simulink library "vs"  (Simulink 5.0)
values from neighbouring files (symbols this model uses):
  RPY = tr2rpy(T0c)    [slidevar.m]
undefined symbols (not defined in the file or in its folder): CamView, ContrLaw
libraries: simulink x24, simulink3 x23, vs x8, vs1 x1
settings Model: LastModifiedBy=ecervera

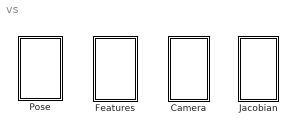
== system vs ==
  Camera : Subsystem
  Features : Subsystem
  Jacobian : Subsystem
  Pose : Subsystem

== system vs/Camera ==
  Camera view : Subsystem  LoadFcn=CamView([],[],[],'LoadBlock')  StartFcn=CamView([],[],[],'Start')  StopFcn=CamView([],[],[],'Stop')  mask{ms=15, em=normal, umin=0, umax=511, vmin=0, vmax=511, st=-1}
      mask prompts: ms "Marker Size"; em "Erase Mode"; st "Sample time"
      settings: CopyFcn=CamView([],[],[],'CopyBlock')  DeleteFcn=CamView([],[],[],'DeleteBlock')  NameChangeFcn=CamView([],[],[],'NameChange')
      mask StyleString: edit,popup(normal|none),edit,edit,edit,edit,edit
  Image of RSP : Subsystem  mask{fu=1, fv=1, u0=0, v0=0}
      mask help: Camera projection of a rigid set of points in camera frame.
  Pose estimation : Subsystem  mask{fu=1000, fv=1000, u0=256, v0=256, threshold=0.001}

== system vs/Features ==
  DTrans : Subsystem
  ITrans : Subsystem
  Penta object : vs/Features/Rigid Set of Points  x=[0 0.25 0.25 -0.25 -0.25]  y=[0 -0.25 0.25 0.25 -0.25]  z=[0 0 0 0 0]
  Point Matrix : Subsystem  mask{m=[]}
      mask prompts: m "Point Matrix (4 x N)"
      mask help: Homogeneous coordinates of a set of 3D points (each point is a matrix column).
  Quad object : vs/Features/Rigid Set of Points  x=[0.25 0.25 -0.25 -0.25]  y=[-0.25 0.25 0.25 -0.25]  z=[0 0 0 0]
  Rigid Set of Points : Subsystem  mask{x=[], y=[], z=[]}
      mask prompts: x "X-vector"; y "Y-vector"; z "Z-vector"
      mask help: Homogeneous coordinates of a set of 3D points (each point is a matrix column).
  Z's of RSP : Subsystem

== system vs/Jacobian ==
  Hand-coded control law : Subsystem  mask{n=5, fu=1000, fv=1000, u0=256, v0=256, lambda=0.125}
      mask prompts: n "Number of points"
  Inverse J : Subsystem
  Jacobian  of 2D points : Subsystem  mask{fu=1000, fv=1000, u0=256, v0=256, lambda=1}
      mask prompts: lambda "Gain"
      mask help: Converts a matrix of pixels (u,v) to a feature vector s of points (x,y) with focal=1.
  Jacobian of 3D points : Subsystem
  Jacobian of RSP : Subsystem
  PBcontrol : Subsystem  mask{lambda=0.05}
      mask prompts: lambda "Gain (>0)"
  PI control law : Subsystem  mask{lambda=1, mu=}
      mask prompts: lambda "Proportional gain (>0)"; mu "Integral gain (>0)"
      mask help: Computes the kinematic screw V = - gain J+ (s - s*).
  Pixel2s : Subsystem  mask{fu=, fv=, u0=, v0=}
      mask help: Converts a matrix of pixels (u,v) to a feature vector s of points (x,y) with focal=1.
  Proportional control law : Subsystem  mask{lambda=1}
      mask prompts: lambda "Gain (>0)"
      mask help: Computes the kinematic screw V = - gain J+ (s - s*).
  Rank J : Subsystem
  Target feature : Subsystem  mask{s=[]}
      mask prompts: s "s*"
      mask help: Column vector of target features: [s1; s2; s3; .... ; sn].
  s for points 3D : Subsystem

== system vs/Pose ==
  Composition : Subsystem
  Frame motion : Subsystem
  Inverse : Subsystem
  Pose : Subsystem  mask{x=0, y=0, z=0, r=RPY, phi=0, theta=0, psi=0}
      mask prompts: r "Rotation"
      mask help: Transformation of a translation + rotation.
      mask StyleString: edit,edit,edit,popup(RPY|Euler),edit,edit,edit
  Pose2Putheta : Subsystem
  Relative : Subsystem
  ScrewTrMat : Subsystem
  ScrewTrans : Subsystem
  skew-sym : Subsystem

== system vs/Camera/Camera view ==
  uv : Inport
  Reshape : simulink3/Signals & Systems/Reshape  OutputDimensionality=1-D array  OutputDimensions=[1,1]
  S-Function : S-Function  FunctionName=CamView  Parameters=[umin umax vmin vmax],st,ms,em
  wires:
  Reshape/1 -> S-Function/1
  uv/1 -> Reshape/1

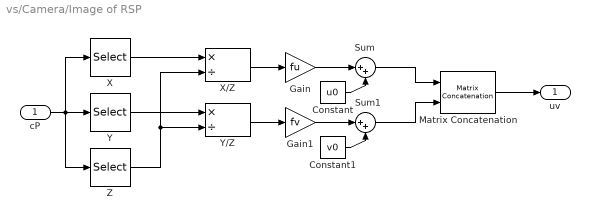
== system vs/Camera/Image of RSP ==
  cP : Inport
  Constant : Constant  Value=u0
  Constant1 : Constant  Value=v0
  Gain : Gain  Gain=fu  SaturateOnIntegerOverflow=on
  Gain1 : Gain  Gain=fv  SaturateOnIntegerOverflow=on
  Matrix Concatenation : simulink3/Signals & Systems/Matrix Concatenation  numInports=2  catMethod=Vertical
  Sum : Sum  Inputs=|++  SaturateOnIntegerOverflow=on  InputSameDT=on
  Sum1 : Sum  Inputs=|++  SaturateOnIntegerOverflow=on  InputSameDT=on
  X : Selector  InputType=Matrix  Elements=[1 3]  Columns=-1  InputPortWidth=3
  X/Z : Product  Inputs=*/  SaturateOnIntegerOverflow=on  InputSameDT=on
  Y : Selector  InputType=Matrix  Elements=[1 3]  Rows=2  Columns=-1  InputPortWidth=3
  Y/Z : Product  Inputs=*/  SaturateOnIntegerOverflow=on  InputSameDT=on
  Z : Selector  InputType=Matrix  Elements=[1 3]  Rows=3  Columns=-1  InputPortWidth=3
  uv : Outport
  wires:
  cP/1 -> X/1, Y/1, Z/1
  X/1 -> X/Z/1
  Z/1 -> X/Z/2, Y/Z/2
  Y/1 -> Y/Z/1
  Y/Z/1 -> Gain1/1
  X/Z/1 -> Gain/1
  Gain/1 -> Sum/1
  Gain1/1 -> Sum1/1
  Constant/1 -> Sum/2
  Constant1/1 -> Sum1/2
  Sum/1 -> Matrix Concatenation/1
  Sum1/1 -> Matrix Concatenation/2
  Matrix Concatenation/1 -> uv/1

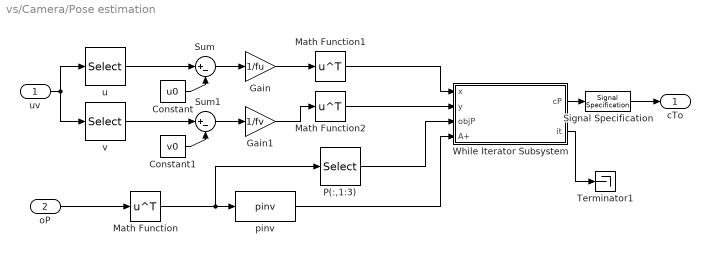
== system vs/Camera/Pose estimation ==
  uv : Inport
  oP : Inport  Port=2
  Constant : Constant  Value=u0
  Constant1 : Constant  Value=v0
  Gain : Gain  Gain=1/fu  SaturateOnIntegerOverflow=on
  Gain1 : Gain  Gain=1/fv  SaturateOnIntegerOverflow=on
  Math Function : Math  Operator=transpose
  Math Function1 : Math  Operator=transpose
  Math Function2 : Math  Operator=transpose
  P(:,1:3) : Selector  InputType=Matrix  Elements=[1 3]  Rows=-1  Columns=[1 2 3]  InputPortWidth=3
  Signal Specification : simulink/Signal Attributes/Signal Specification  D=[4 4]  Ts=-1  DataType=auto  OutDataType=sfix(16)  OutScaling=2^0
      settings: SignalType=auto  SamplingMode=auto
  Sum : Sum  Inputs=|+-  SaturateOnIntegerOverflow=on  InputSameDT=on
  Sum1 : Sum  Inputs=|+-  SaturateOnIntegerOverflow=on  InputSameDT=on
  Terminator1 : Terminator
  While Iterator Subsystem : Subsystem  TreatAsAtomicUnit=on
  pinv : MATLABFcn  MATLABFcn=pinv  Output1D=off
  u : Selector  InputType=Matrix  Elements=[1 3]  Columns=-1  InputPortWidth=3
  v : Selector  InputType=Matrix  Elements=[1 3]  Rows=2  Columns=-1  InputPortWidth=3
  cTo : Outport
  wires:
  While Iterator Subsystem/1(cP) -> Signal Specification/1
  uv/1 -> u/1, v/1
  u/1 -> Sum/1
  v/1 -> Sum1/1
  Constant/1 -> Sum/2
  Constant1/1 -> Sum1/2
  Sum/1 -> Gain/1
  Sum1/1 -> Gain1/1
  Gain/1 -> Math Function1/1
  Gain1/1 -> Math Function2/1
  oP/1 -> Math Function/1
  Math Function/1 -> pinv/1, P(:,1:3)/1
  Math Function1/1 -> While Iterator Subsystem/1(x)
  pinv/1 -> While Iterator Subsystem/4(A+)
  Math Function2/1 -> While Iterator Subsystem/2(y)
  P(:,1:3)/1 -> While Iterator Subsystem/3(objP)
  While Iterator Subsystem/2(it) -> Terminator1/1
  Signal Specification/1 -> cTo/1

== system vs/Features/DTrans ==
  aTb : Inport
  bP : Inport  Port=2
  Product : Product  Multiplication=Matrix(*)  SaturateOnIntegerOverflow=on  InputSameDT=on
  aP : Outport
  wires:
  aTb/1 -> Product/1
  bP/1 -> Product/2
  Product/1 -> aP/1

== system vs/Features/ITrans ==
  aTb : Inport
  aP : Inport  Port=2
  Inverse : vs/Pose/Inverse
      settings: RTWFcnNameOpts=Auto  RTWFileNameOpts=Auto
  Product : Product  Multiplication=Matrix(*)  SaturateOnIntegerOverflow=on  InputSameDT=on
  bP : Outport
  wires:
  aP/1 -> Product/2
  Product/1 -> bP/1
  aTb/1 -> Inverse/1
  Inverse/1 -> Product/1

== system vs/Features/Point Matrix ==
  Constant : Constant  Value=m  VectorParams1D=off
  P : Outport
  wires:
  Constant/1 -> P/1

== system vs/Features/Rigid Set of Points ==
  Constant : Constant  Value=[x;y;z;ones(1,length(x))]  VectorParams1D=off
  P : Outport
  wires:
  Constant/1 -> P/1

== system vs/Features/Z's of RSP ==
  P : Inport
  Math Function : Math  Operator=transpose
  Select Z : Selector  InputType=Matrix  Elements=[1 3]  Rows=3  Columns=-1  InputPortWidth=3
  Z : Outport
  wires:
  P/1 -> Select Z/1
  Select Z/1 -> Math Function/1
  Math Function/1 -> Z/1

== system vs/Jacobian/Hand-coded control law ==
  uv : Inport
  Z : Inport  Port=2
  uv* : Inport  Port=3
  MATLAB Fcn : MATLABFcn  MATLABFcn=ContrLaw(reshape(u(1:2*n),2,n),u(2*n+1:3*n),reshape(u(3*n+1:5*n),2,n),fu,fv,u0,v0,lambda)  OutputDimensions=6  Output1D=off
  Mux : Mux  Inputs=3
  Reshape : simulink3/Signals & Systems/Reshape  OutputDimensionality=1-D array  OutputDimensions=[1,1]
  Reshape1 : simulink3/Signals & Systems/Reshape  OutputDimensionality=1-D array  OutputDimensions=[1,1]
  Reshape2 : simulink3/Signals & Systems/Reshape  OutputDimensionality=1-D array  OutputDimensions=[1,1]
  Reshape3 : simulink3/Signals & Systems/Reshape  OutputDimensionality=Column vector  OutputDimensions=[1,1]
  cVc : Outport
  wires:
  MATLAB Fcn/1 -> Reshape3/1
  uv/1 -> Reshape/1
  Z/1 -> Reshape1/1
  uv*/1 -> Reshape2/1
  Mux/1 -> MATLAB Fcn/1
  Reshape/1 -> Mux/1
  Reshape1/1 -> Mux/2
  Reshape2/1 -> Mux/3
  Reshape3/1 -> cVc/1

== system vs/Jacobian/Inverse J ==
  J : Inport
  pinv : MATLABFcn  MATLABFcn=pinv  Output1D=off
  J+ : Outport
  wires:
  J/1 -> pinv/1
  pinv/1 -> J+/1

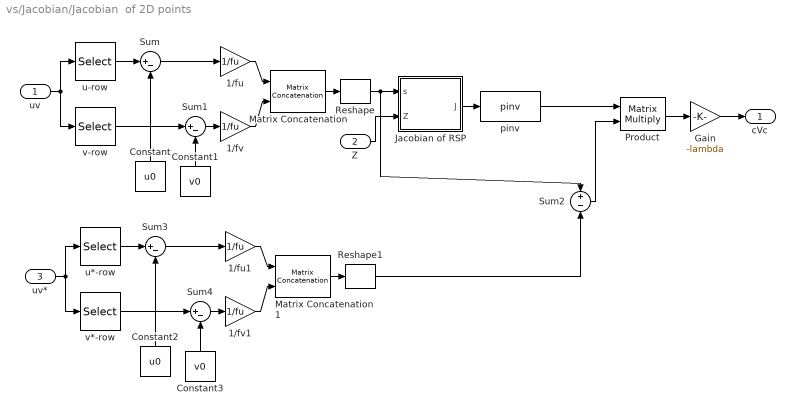
== system vs/Jacobian/Jacobian  of 2D points ==
  uv : Inport
  Z : Inport  Port=2
  uv* : Inport  Port=3
  1/fu : Gain  Gain=1/fu  SaturateOnIntegerOverflow=on
  1/fu1 : Gain  Gain=1/fu  SaturateOnIntegerOverflow=on
  1/fv : Gain  Gain=1/fu  SaturateOnIntegerOverflow=on
  1/fv1 : Gain  Gain=1/fu  SaturateOnIntegerOverflow=on
  Constant : Constant  Orientation=up  Value=u0
  Constant1 : Constant  Orientation=up  Value=v0
  Constant2 : Constant  Orientation=up  Value=u0
  Constant3 : Constant  Orientation=up  Value=v0
  Gain : Gain  Gain=-lambda  SaturateOnIntegerOverflow=on
  Jacobian of RSP : Subsystem
  Matrix Concatenation : simulink3/Signals & Systems/Matrix Concatenation  numInports=2  catMethod=Vertical
  Matrix Concatenation1 : simulink3/Signals & Systems/Matrix Concatenation  numInports=2  catMethod=Vertical
  Product : Product  Multiplication=Matrix(*)  SaturateOnIntegerOverflow=on  InputSameDT=on
  Reshape : simulink3/Signals & Systems/Reshape  OutputDimensionality=Column vector  OutputDimensions=[1,1]
  Reshape1 : simulink3/Signals & Systems/Reshape  OutputDimensionality=Column vector  OutputDimensions=[1,1]
  Sum{,1,3..4} (4 alike) : Sum  Inputs=|+-  SaturateOnIntegerOverflow=on  InputSameDT=on
  Sum2 : Sum  Inputs=+-  SaturateOnIntegerOverflow=on  InputSameDT=on
  pinv : MATLABFcn  MATLABFcn=pinv  Output1D=off
  u*-row : Selector  InputType=Matrix  Elements=[1 3]  Columns=-1  InputPortWidth=3
  u-row : Selector  InputType=Matrix  Elements=[1 3]  Columns=-1  InputPortWidth=3
  v*-row : Selector  InputType=Matrix  Elements=[1 3]  Rows=2  Columns=-1  InputPortWidth=3
  v-row : Selector  InputType=Matrix  Elements=[1 3]  Rows=2  Columns=-1  InputPortWidth=3
  cVc : Outport
  wires:
  Reshape/1 -> Jacobian of RSP/1(s), Sum2/1
  uv/1 -> v-row/1, u-row/1
  u-row/1 -> Sum/1
  v-row/1 -> Sum1/1
  Sum/1 -> 1/fu/1
  Sum1/1 -> 1/fv/1
  1/fu/1 -> Matrix Concatenation/1
  1/fv/1 -> Matrix Concatenation/2
  Matrix Concatenation/1 -> Reshape/1
  Constant/1 -> Sum/2
  Constant1/1 -> Sum1/2
  Z/1 -> Jacobian of RSP/2(Z)
  Jacobian of RSP/1(J) -> pinv/1
  Sum2/1 -> Product/2
  Product/1 -> Gain/1
  Gain/1 -> cVc/1
  pinv/1 -> Product/1
  uv*/1 -> v*-row/1, u*-row/1
  u*-row/1 -> Sum3/1
  v*-row/1 -> Sum4/1
  Sum3/1 -> 1/fu1/1
  Sum4/1 -> 1/fv1/1
  1/fu1/1 -> Matrix Concatenation1/1
  1/fv1/1 -> Matrix Concatenation1/2
  Matrix Concatenation1/1 -> Reshape1/1
  Constant2/1 -> Sum3/2
  Constant3/1 -> Sum4/2
  Reshape1/1 -> Sum2/2

== system vs/Jacobian/Jacobian of 3D points ==
  s : Inport
  Constant : Constant  Value=3
  Jacobian stack : Subsystem  TreatAsAtomicUnit=on
  Product : Product  Inputs=*/  SaturateOnIntegerOverflow=on  InputSameDT=on
  Width : Width
  J : Outport
  wires:
  Jacobian stack/1(J) -> J/1
  s/1 -> Jacobian stack/1(s), Width/1
  Product/1 -> Jacobian stack/2(n)
  Width/1 -> Product/1
  Constant/1 -> Product/2

== system vs/Jacobian/Jacobian of RSP ==
  s : Inport
  Z : Inport  Port=2
  Jacobian stack : Subsystem  TreatAsAtomicUnit=on
  Width : Width
  J : Outport
  wires:
  Jacobian stack/1(J) -> J/1
  s/1 -> Jacobian stack/1(s)
  Width/1 -> Jacobian stack/3(n)
  Z/1 -> Width/1, Jacobian stack/2(Z)

== system vs/Jacobian/PBcontrol ==
  P : Inport
  u : Inport  Port=2
  theta : Inport  Port=3
  Gain : Gain  Gain=lambda  SaturateOnIntegerOverflow=on
  Matrix Concatenation : simulink3/Signals & Systems/Matrix Concatenation  numInports=2  catMethod=Vertical
  Product : Product  SaturateOnIntegerOverflow=on  InputSameDT=on
  cVc : Outport
  wires:
  Product/1 -> Matrix Concatenation/2
  Matrix Concatenation/1 -> Gain/1
  P/1 -> Matrix Concatenation/1
  u/1 -> Product/1
  Gain/1 -> cVc/1
  theta/1 -> Product/2

== system vs/Jacobian/PI control law ==
  J+ : Inport
  s : Inport  Port=2
  s* : Inport  Port=3
  Gain : Gain  Gain=-lambda  SaturateOnIntegerOverflow=on
  Gain1 : Gain  Gain=-mu  SaturateOnIntegerOverflow=on
  Integrator : Integrator
  Product : Product  Multiplication=Matrix(*)  SaturateOnIntegerOverflow=on  InputSameDT=on
  Sum : Sum  Inputs=+-  SaturateOnIntegerOverflow=on  InputSameDT=on
  Sum1 : Sum  Inputs=|++  SaturateOnIntegerOverflow=on  InputSameDT=on
  cVc : Outport
  wires:
  s/1 -> Sum/1
  s*/1 -> Sum/2
  J+/1 -> Product/1
  Sum/1 -> Product/2
  Product/1 -> Gain/1, Integrator/1
  Integrator/1 -> Gain1/1
  Gain/1 -> Sum1/1
  Sum1/1 -> cVc/1
  Gain1/1 -> Sum1/2

== system vs/Jacobian/Pixel2s ==
  uv : Inport
  1/fu : Gain  Gain=1/fu  SaturateOnIntegerOverflow=on
  1/fv : Gain  Gain=1/fu  SaturateOnIntegerOverflow=on
  Constant : Constant  Orientation=up  Value=u0
  Constant1 : Constant  Orientation=up  Value=v0
  Matrix Concatenation : simulink3/Signals & Systems/Matrix Concatenation  numInports=2  catMethod=Vertical
  Reshape : simulink3/Signals & Systems/Reshape  OutputDimensionality=Column vector  OutputDimensions=[1,1]
  Sum : Sum  Inputs=|+-  SaturateOnIntegerOverflow=on  InputSameDT=on
  Sum1 : Sum  Inputs=|+-  SaturateOnIntegerOverflow=on  InputSameDT=on
  u-row : Selector  InputType=Matrix  Elements=[1 3]  Columns=-1  InputPortWidth=3
  v-row : Selector  InputType=Matrix  Elements=[1 3]  Rows=2  Columns=-1  InputPortWidth=3
  s : Outport
  wires:
  Reshape/1 -> s/1
  uv/1 -> v-row/1, u-row/1
  u-row/1 -> Sum/1
  v-row/1 -> Sum1/1
  Sum/1 -> 1/fu/1
  Sum1/1 -> 1/fv/1
  1/fu/1 -> Matrix Concatenation/1
  1/fv/1 -> Matrix Concatenation/2
  Matrix Concatenation/1 -> Reshape/1
  Constant/1 -> Sum/2
  Constant1/1 -> Sum1/2

== system vs/Jacobian/Proportional control law ==
  J+ : Inport
  s : Inport  Port=2
  s* : Inport  Port=3
  Gain : Gain  Gain=-lambda  SaturateOnIntegerOverflow=on
  Product : Product  Multiplication=Matrix(*)  SaturateOnIntegerOverflow=on  InputSameDT=on
  Sum : Sum  Inputs=+-  SaturateOnIntegerOverflow=on  InputSameDT=on
  cVc : Outport
  wires:
  s/1 -> Sum/1
  s*/1 -> Sum/2
  J+/1 -> Product/1
  Sum/1 -> Product/2
  Product/1 -> Gain/1
  Gain/1 -> cVc/1

== system vs/Jacobian/Rank J ==
  J : Inport
  rank : MATLABFcn  MATLABFcn=rank  Output1D=off
  Rank(J) : Outport
  wires:
  J/1 -> rank/1
  rank/1 -> Rank(J)/1

== system vs/Jacobian/Target feature ==
  Constant : Constant  Value=s  VectorParams1D=off
  s* : Outport
  wires:
  Constant/1 -> s*/1

== system vs/Jacobian/s for points 3D ==
  cP : Inport
  Reshape : simulink3/Signals & Systems/Reshape  OutputDimensionality=Column vector  OutputDimensions=[1,1]
  Selector : Selector  InputType=Matrix  Elements=[1 3]  Rows=[1 2 3]  Columns=-1  InputPortWidth=3
  s : Outport
  wires:
  cP/1 -> Selector/1
  Reshape/1 -> s/1
  Selector/1 -> Reshape/1

== system vs/Pose/Composition ==
  aTb : Inport
  bTc : Inport  Port=2
  Product : Product  Multiplication=Matrix(*)  SaturateOnIntegerOverflow=on  InputSameDT=on
  aTc : Outport
  wires:
  Product/1 -> aTc/1
  aTb/1 -> Product/1
  bTc/1 -> Product/2

== system vs/Pose/Frame motion ==
  iTj(0) : Inport
  jVj : Inport  Port=2
  Differential : Subsystem
  Motion : Subsystem
  iTj(t) : Outport
  wires:
  Differential/1(diTj) -> Motion/2(diTj)
  iTj(0)/1 -> Motion/1(iTj(0))
  Motion/1(iTj(t)) -> iTj(t)/1, Differential/1(iTj)
  jVj/1 -> Differential/2(Vj)

== system vs/Pose/Inverse ==
  aTb : Inport
  Math Function : Math  Operator=transpose
  Matrix Gain : Gain  Gain=[1 0 0 0; 0 1 0 0; 0 0 1 0; 0 0 0 -1]  Multiplication=Matrix(u*K)  SaturateOnIntegerOverflow=on
  Matrix Gain1 : Gain  Gain=[1 0 0 0; 0 1 0 0; 0 0 1 0; 0 0 0 -1]  Multiplication=Matrix(u*K)  SaturateOnIntegerOverflow=on
  Product1 : Product  Multiplication=Matrix(*)  SaturateOnIntegerOverflow=on  InputSameDT=on
  Split : Subsystem
  bTa : Outport
  wires:
  aTb/1 -> Split/1(T)
  Split/1(R) -> Math Function/1
  Product1/1 -> bTa/1
  Matrix Gain/1 -> Product1/2
  Split/2(P) -> Matrix Gain/1
  Matrix Gain1/1 -> Product1/1
  Math Function/1 -> Matrix Gain1/1

== system vs/Pose/Pose ==
  Constant : Constant  Value=r
  Euler-rotation : Subsystem  mask{phi=phi, theta=theta, psi=psi}
      mask help: Transformation of a rotation specified by Euler angles: T = rot(z,phi) rot(x,theta) rot(z, psi).
  Product : Product  Multiplication=Matrix(*)  SaturateOnIntegerOverflow=on  InputSameDT=on
  RPY-rotation : Subsystem  mask{phi=phi, theta=theta, psi=psi}
      mask help: Transformation of a rotation specified by Euler angles: T = rot(z,phi) rot(x,theta) rot(z, psi).
  Switch : Switch  Threshold=1.5  SaturateOnIntegerOverflow=on  InputSameDT=on
  Translation : Subsystem  mask{x=x, y=y, z=z}
      mask help: Transformation of a pure translation.
  T : Outport
  wires:
  Euler-rotation/1(T) -> Switch/1
  RPY-rotation/1(T) -> Switch/3
  Constant/1 -> Switch/2
  Product/1 -> T/1
  Translation/1(T) -> Product/1
  Switch/1 -> Product/2

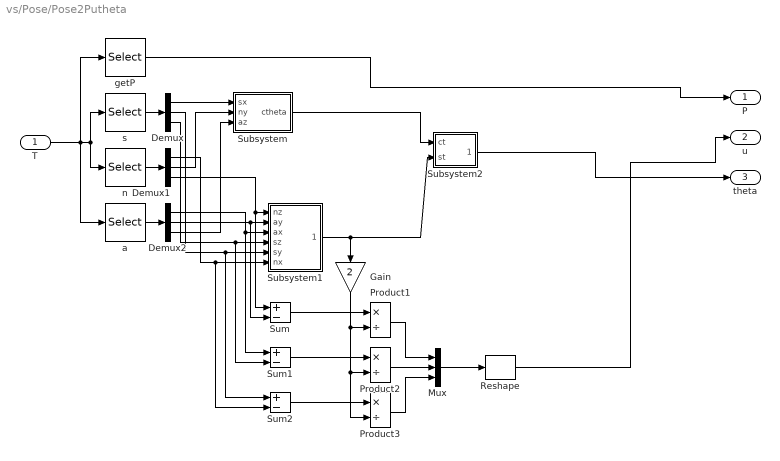
== system vs/Pose/Pose2Putheta ==
  T : Inport
  Demux : Demux  Outputs=3
  Demux1 : Demux  Outputs=3
  Demux2 : Demux  Outputs=3
  Gain : Gain  Orientation=down  Gain=2  SaturateOnIntegerOverflow=on
  Mux : Mux  Inputs=3
  Product1 : Product  Inputs=*/  SaturateOnIntegerOverflow=on  InputSameDT=on
  Product2 : Product  Inputs=*/  SaturateOnIntegerOverflow=on  InputSameDT=on
  Product3 : Product  Inputs=*/  SaturateOnIntegerOverflow=on  InputSameDT=on
  Reshape : simulink3/Signals & Systems/Reshape  OutputDimensionality=Column vector  OutputDimensions=[1,1]
  Subsystem : Subsystem
  Subsystem1 : Subsystem
  Subsystem2 : Subsystem
  Sum : Sum  Inputs=+-  SaturateOnIntegerOverflow=on  InputSameDT=on
  Sum1 : Sum  Inputs=+-  SaturateOnIntegerOverflow=on  InputSameDT=on
  Sum2 : Sum  Inputs=+-  SaturateOnIntegerOverflow=on  InputSameDT=on
  a : Selector  InputType=Matrix  Elements=[1 3]  Rows=[1 2 3]  Columns=3  InputPortWidth=3
  getP : Selector  InputType=Matrix  Elements=[1 3]  Rows=[1 2 3]  Columns=4  InputPortWidth=3
  n : Selector  InputType=Matrix  Elements=[1 3]  Rows=[1 2 3]  Columns=2  InputPortWidth=3
  s : Selector  InputType=Matrix  Elements=[1 3]  Rows=[1 2 3]  InputPortWidth=3
  P : Outport
  u : Outport  Port=2
  theta : Outport  Port=3
  wires:
  T/1 -> getP/1, s/1, n/1, a/1
  getP/1 -> P/1
  s/1 -> Demux/1
  n/1 -> Demux1/1
  a/1 -> Demux2/1
  Demux/1 -> Subsystem/1(sx)
  Demux1/2 -> Subsystem/2(ny)
  Demux2/3 -> Subsystem/3(az)
  Demux1/3 -> Subsystem1/1(nz), Sum/1
  Demux2/2 -> Subsystem1/2(ay), Sum/2
  Demux2/1 -> Subsystem1/3(ax), Sum1/1
  Demux/3 -> Subsystem1/4(sz), Sum1/2
  Demux/2 -> Subsystem1/5(sy), Sum2/1
  Demux1/1 -> Subsystem1/6(nx), Sum2/2
  Subsystem/1(ctheta) -> Subsystem2/1(ct)
  Subsystem1/1(stheta) -> Subsystem2/2(st), Gain/1
  Gain/1 -> Product1/2, Product2/2, Product3/2
  Sum/1 -> Product1/1
  Sum1/1 -> Product2/1
  Sum2/1 -> Product3/1
  Product2/1 -> Mux/2
  Product1/1 -> Mux/1
  Product3/1 -> Mux/3
  Subsystem2/1(theta) -> theta/1
  Mux/1 -> Reshape/1
  Reshape/1 -> u/1

== system vs/Pose/Relative ==
  aTb : Inport
  aTc : Inport  Port=2
  Inverse : vs1/Pose/Inverse
      settings: RTWFcnNameOpts=Auto  RTWFileNameOpts=Auto
  Product : Product  Multiplication=Matrix(*)  SaturateOnIntegerOverflow=on  InputSameDT=on
  bTc : Outport
  wires:
  Product/1 -> bTc/1
  aTb/1 -> Inverse/1
  Inverse/1 -> Product/1
  aTc/1 -> Product/2

== system vs/Pose/ScrewTrMat ==
  iTj : Inport
  0 3x3 : Constant  Value=zeros(3,3)  VectorParams1D=off
  Matrix Concatenation : simulink/Math Operations/Matrix Concatenation  numInports=2  catMethod=Horizontal
  Matrix Concatenation1 : simulink/Math Operations/Matrix Concatenation  numInports=2  catMethod=Horizontal
  Matrix Concatenation2 : simulink/Math Operations/Matrix Concatenation  numInports=2  catMethod=Vertical
  Product : Product  Multiplication=Matrix(*)  SaturateOnIntegerOverflow=on  InputSameDT=on
  Split : Subsystem
  iPj 3x1 : Selector  InputType=Matrix  Elements=[1 3]  Rows=[1 2 3]  Columns=4  InputPortWidth=3
  iRj 3x3 : Selector  InputType=Matrix  Elements=[1 3]  Rows=[1 2 3]  Columns=[1 2 3]  InputPortWidth=3
  sk(iPj) : vs/Pose/skew-sym  SimViewingDevice=off  DataTypeOverride=UseLocalSettings  MinMaxOverflowLogging=UseLocalSettings
      settings: Permissions=ReadWrite  RTWFcnNameOpts=Auto  RTWFileNameOpts=Auto
  iSTj : Outport
  wires:
  0 3x3/1 -> Matrix Concatenation1/1
  sk(iPj)/1 -> Product/1
  Product/1 -> Matrix Concatenation/2
  iRj 3x3/1 -> Matrix Concatenation1/2, Product/2, Matrix Concatenation/1
  Matrix Concatenation1/1 -> Matrix Concatenation2/2
  Matrix Concatenation/1 -> Matrix Concatenation2/1
  Matrix Concatenation2/1 -> iSTj/1
  iPj 3x1/1 -> sk(iPj)/1
  Split/2(P) -> iPj 3x1/1
  Split/1(R) -> iRj 3x3/1
  iTj/1 -> Split/1(T)

== system vs/Pose/ScrewTrans ==
  jVj : Inport
  iTj : Inport  Port=2
  Product : Product  Multiplication=Matrix(*)  SaturateOnIntegerOverflow=on  InputSameDT=on
  ScrewTrMat : vs/Pose/ScrewTrMat  SimViewingDevice=off  DataTypeOverride=UseLocalSettings  MinMaxOverflowLogging=UseLocalSettings
      settings: Permissions=ReadWrite  RTWFcnNameOpts=Auto  RTWFileNameOpts=Auto
  iVi : Outport
  wires:
  iTj/1 -> ScrewTrMat/1
  ScrewTrMat/1 -> Product/1
  jVj/1 -> Product/2
  Product/1 -> iVi/1

== system vs/Pose/skew-sym ==
  v : Inport
  Constant : Constant  Value=[0 0 0; 0 0 1; 0 -1 0]  VectorParams1D=off
  Constant1 : Constant  Value=[0 0 -1; 0 0 0; 1 0 0]  VectorParams1D=off
  Constant2 : Constant  Value=[0 1 0; -1 0 0; 0 0 0]  VectorParams1D=off
  Matrix Concatenation : simulink/Math Operations/Matrix Concatenation  numInports=3  catMethod=Horizontal
  Product : Product  Multiplication=Matrix(*)  SaturateOnIntegerOverflow=on  InputSameDT=on
  Product1 : Product  Multiplication=Matrix(*)  SaturateOnIntegerOverflow=on  InputSameDT=on
  Product2 : Product  Multiplication=Matrix(*)  SaturateOnIntegerOverflow=on  InputSameDT=on
  Signal Specification1 : simulink/Signal Attributes/Signal Specification  D=[3 1]  Ts=-1  DataType=auto  OutDataType=sfix(16)  OutScaling=2^0
      settings: SignalType=auto  SamplingMode=auto
  Signal Specification2 : simulink/Signal Attributes/Signal Specification  D=[3 1]  Ts=-1  DataType=auto  OutDataType=sfix(16)  OutScaling=2^0
      settings: SignalType=auto  SamplingMode=auto
  Signal Specification3 : simulink/Signal Attributes/Signal Specification  D=[3 1]  Ts=-1  DataType=auto  OutDataType=sfix(16)  OutScaling=2^0
      settings: SignalType=auto  SamplingMode=auto
  sk(v) : Outport
  wires:
  Signal Specification3/1 -> Matrix Concatenation/3
  Signal Specification2/1 -> Matrix Concatenation/1
  Signal Specification1/1 -> Matrix Concatenation/2
  Constant/1 -> Product/1
  v/1 -> Product/2, Product1/2, Product2/2
  Matrix Concatenation/1 -> sk(v)/1
  Product/1 -> Signal Specification2/1
  Constant1/1 -> Product1/1
  Constant2/1 -> Product2/1
  Product1/1 -> Signal Specification1/1
  Product2/1 -> Signal Specification3/1

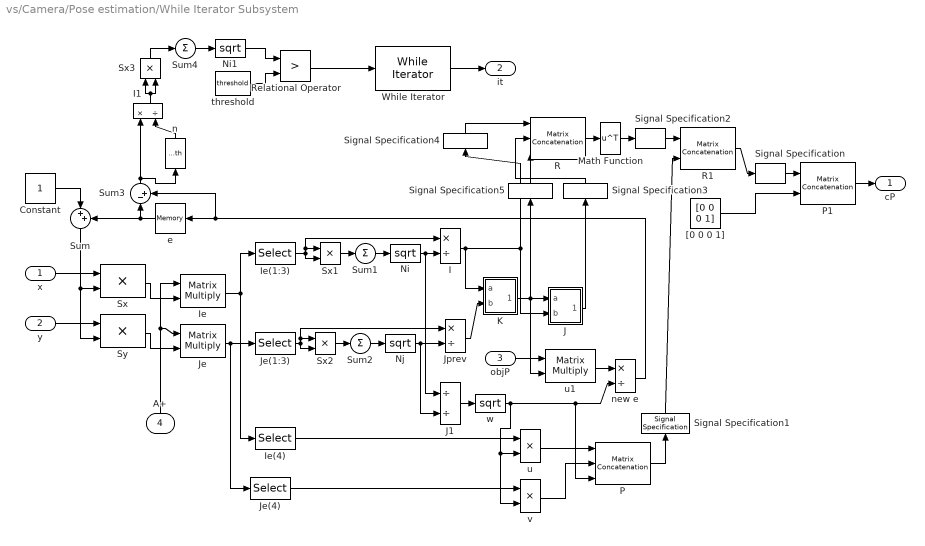
== system vs/Camera/Pose estimation/While Iterator Subsystem ==
  x : Inport
  y : Inport  Port=2
  objP : Inport  Port=3
  A+ : Inport  Orientation=up  Port=4
  Constant : Constant
  I : Product  Inputs=*/  SaturateOnIntegerOverflow=on  InputSameDT=on
  I1 : Product  Orientation=up  Inputs=*/  SaturateOnIntegerOverflow=on  InputSameDT=on
  Ie : Product  Multiplication=Matrix(*)  SaturateOnIntegerOverflow=on  InputSameDT=on
  Ie(1:3) : Selector  InputType=Matrix  Elements=[1 3]  Rows=[1 2 3]  Columns=-1  InputPortWidth=3
  Ie(4) : Selector  InputType=Matrix  Elements=[1 3]  Rows=4  Columns=-1  InputPortWidth=3
  J : Subsystem
  J1 : Product  Inputs=//  SaturateOnIntegerOverflow=on  InputSameDT=on
  Je : Product  Multiplication=Matrix(*)  SaturateOnIntegerOverflow=on  InputSameDT=on
  Je(1:3) : Selector  InputType=Matrix  Elements=[1 3]  Rows=[1 2 3]  Columns=-1  InputPortWidth=3
  Je(4) : Selector  InputType=Matrix  Elements=[1 3]  Rows=4  Columns=-1  InputPortWidth=3
  Jprev : Product  Inputs=*/  SaturateOnIntegerOverflow=on  InputSameDT=on
  K : Subsystem
  Math Function : Math  Operator=transpose
  Ni : Math  Operator=sqrt
  Ni1 : Math  Operator=sqrt
  Nj : Math  Operator=sqrt
  P : simulink/Math Operations/Matrix Concatenation  numInports=3  catMethod=Vertical
  P1 : simulink/Math Operations/Matrix Concatenation  numInports=2  catMethod=Vertical
  R : simulink/Math Operations/Matrix Concatenation  numInports=3  catMethod=Horizontal
  R1 : simulink/Math Operations/Matrix Concatenation  numInports=2  catMethod=Horizontal
  Relational Operator : RelationalOperator  Operator=>  InputSameDT=on
  Signal Specification : simulink/Signal Attributes/Signal Specification  D=[3 4]  Ts=-1  DataType=auto  OutDataType=sfix(16)  OutScaling=2^0
      settings: SignalType=auto  SamplingMode=auto
  Signal Specification{1,3..5} (4 alike) : simulink/Signal Attributes/Signal Specification  Orientation=up  D=[3 1]  Ts=-1  DataType=auto  OutDataType=sfix(16)  OutScaling=2^0
      settings: SignalType=auto  SamplingMode=auto
  Signal Specification2 : simulink/Signal Attributes/Signal Specification  D=[3 3]  Ts=-1  DataType=auto  OutDataType=sfix(16)  OutScaling=2^0
      settings: SignalType=auto  SamplingMode=auto
  Sum : Sum  Orientation=down  Inputs=|++  SaturateOnIntegerOverflow=on  InputSameDT=on
  Sum1 : Sum  Inputs=+  SaturateOnIntegerOverflow=on  InputSameDT=on
  Sum2 : Sum  Inputs=+  SaturateOnIntegerOverflow=on  InputSameDT=on
  Sum3 : Sum  Orientation=up  Inputs=|-+  SaturateOnIntegerOverflow=on  InputSameDT=on
  Sum4 : Sum  Inputs=+  SaturateOnIntegerOverflow=on  InputSameDT=on
  Sx : Product  SaturateOnIntegerOverflow=on  InputSameDT=on
  Sx1 : Product  SaturateOnIntegerOverflow=on  InputSameDT=on
  Sx2 : Product  SaturateOnIntegerOverflow=on  InputSameDT=on
  Sx3 : Product  Orientation=up  SaturateOnIntegerOverflow=on  InputSameDT=on
  Sy : Product  SaturateOnIntegerOverflow=on  InputSameDT=on
  While Iterator : WhileIterator  MaxIters=20  WhileBlockType=do-while  ShowIterationPort=on  OutputDataType=double
  "[0 0 0 1]" : Constant  Value=[0 0 0 1]  VectorParams1D=off
  e : Memory  Orientation=left  InheritSampleTime=on
  n : Width  Orientation=up
  new e : Product  Inputs=*/  SaturateOnIntegerOverflow=on  InputSameDT=on
  threshold : Constant  Value=threshold
  u : Product  Inputs=**  SaturateOnIntegerOverflow=on  InputSameDT=on
  u1 : Product  Inputs=**  Multiplication=Matrix(*)  SaturateOnIntegerOverflow=on  InputSameDT=on
  v : Product  Inputs=**  SaturateOnIntegerOverflow=on  InputSameDT=on
  w : Math  Operator=sqrt
  cP : Outport
  it : Outport  Port=2
  wires:
  x/1 -> Sx/1
  Constant/1 -> Sum/1
  Sum/1 -> Sx/2, Sy/2
  y/1 -> Sy/1
  A+/1 -> Ie/1, Je/1
  Ie/1 -> Ie(4)/1, Ie(1:3)/1
  Je/1 -> Je(1:3)/1, Je(4)/1
  Ie(1:3)/1 -> Sx1/2, Sx1/1, I/1
  Sx1/1 -> Sum1/1
  Sum1/1 -> Ni/1
  Je(1:3)/1 -> Sx2/2, Sx2/1, Jprev/1
  Sx2/1 -> Sum2/1
  Sum2/1 -> Nj/1
  Ni/1 -> I/2, J1/1
  Nj/1 -> Jprev/2, J1/2
  I/1 -> K/1(a), J/2(b), Signal Specification4/1
  Jprev/1 -> K/2(b)
  K/1(axb) -> J/1(a), u1/2, Signal Specification5/1
  J1/1 -> w/1
  Ie(4)/1 -> u/1
  w/1 -> u/2, v/2, new e/2, P/3
  Je(4)/1 -> v/1
  objP/1 -> u1/1
  u1/1 -> new e/1
  e/1 -> Sum/2, Sum3/1
  new e/1 -> e/1, Sum3/2
  Sum3/1 -> n/1, I1/1
  n/1 -> I1/2
  I1/1 -> Sx3/1, Sx3/2
  Sx3/1 -> Sum4/1
  Sum4/1 -> Ni1/1
  Ni1/1 -> Relational Operator/1
  threshold/1 -> Relational Operator/2
  Relational Operator/1 -> While Iterator/1
  While Iterator/1 -> it/1
  J/1(axb) -> Signal Specification3/1
  u/1 -> P/1
  v/1 -> P/2
  R/1 -> Math Function/1
  P/1 -> Signal Specification1/1
  R1/1 -> Signal Specification/1
  P1/1 -> cP/1
  Sx/1 -> Ie/2
  Sy/1 -> Je/2
  Math Function/1 -> Signal Specification2/1
  "[0 0 0 1]"/1 -> P1/2
  Signal Specification/1 -> P1/1
  Signal Specification1/1 -> R1/2
  Signal Specification2/1 -> R1/1
  Signal Specification3/1 -> R/2
  Signal Specification4/1 -> R/1
  Signal Specification5/1 -> R/3

== system vs/Jacobian/Jacobian  of 2D points/Jacobian of RSP ==
  s : Inport
  Z : Inport  Port=2
  Jacobian stack : Subsystem  TreatAsAtomicUnit=on
  Width : Width
  J : Outport
  wires:
  Jacobian stack/1(J) -> J/1
  s/1 -> Jacobian stack/1(s)
  Width/1 -> Jacobian stack/3(n)
  Z/1 -> Width/1, Jacobian stack/2(Z)

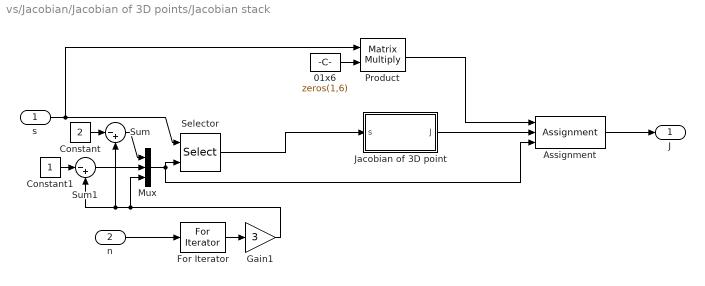
== system vs/Jacobian/Jacobian of 3D points/Jacobian stack ==
  s : Inport
  n : Inport  Port=2
  01x6 : Constant  Value=zeros(1,6)  VectorParams1D=off
  Assignment : Assignment  InputType=Matrix  RowSrc=External  Columns=-1
  Constant : Constant  Value=2
  Constant1 : Constant
  For Iterator : ForIterator  IterationSource=external  OutputDataType=double
  Gain1 : Gain  Gain=3  SaturateOnIntegerOverflow=on
  Jacobian of 3D point : Subsystem
  Mux : Mux  Inputs=3
  Product : Product  Multiplication=Matrix(*)  SaturateOnIntegerOverflow=on  InputSameDT=on
  Selector : Selector  InputType=Matrix  ElementSrc=External  Elements=[1 3]  RowSrc=External  Columns=-1  InputPortWidth=3
  Sum : Sum  Inputs=|-+  SaturateOnIntegerOverflow=on  InputSameDT=on
  Sum1 : Sum  Inputs=|-+  SaturateOnIntegerOverflow=on  InputSameDT=on
  J : Outport
  wires:
  Selector/1 -> Jacobian of 3D point/1(s)
  Jacobian of 3D point/1(J) -> Assignment/2
  Constant/1 -> Sum/1
  Sum/1 -> Mux/1
  Gain1/1 -> Mux/3, Sum/2, Sum1/2
  For Iterator/1 -> Gain1/1
  Mux/1 -> Assignment/3, Selector/2
  01x6/1 -> Product/2
  Product/1 -> Assignment/1
  Assignment/1 -> J/1
  n/1 -> For Iterator/1
  s/1 -> Selector/1, Product/1
  Constant1/1 -> Sum1/1
  Sum1/1 -> Mux/2

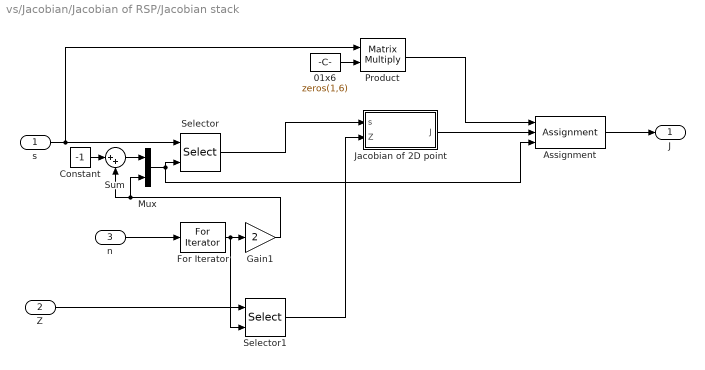
== system vs/Jacobian/Jacobian of RSP/Jacobian stack ==
  s : Inport
  Z : Inport  Port=2
  n : Inport  Port=3
  01x6 : Constant  Value=zeros(1,6)  VectorParams1D=off
  Assignment : Assignment  InputType=Matrix  RowSrc=External  Columns=-1
  Constant : Constant  Value=-1
  For Iterator : ForIterator  IterationSource=external  OutputDataType=double
  Gain1 : Gain  Gain=2  SaturateOnIntegerOverflow=on
  Jacobian of 2D point : Subsystem
  Mux : Mux  Inputs=2
  Product : Product  Multiplication=Matrix(*)  SaturateOnIntegerOverflow=on  InputSameDT=on
  Selector : Selector  InputType=Matrix  ElementSrc=External  Elements=[1 3]  RowSrc=External  Columns=-1  InputPortWidth=3
  Selector1 : Selector  InputType=Matrix  ElementSrc=External  Elements=[1 3]  RowSrc=External  Columns=-1  InputPortWidth=3
  Sum : Sum  Inputs=|++  SaturateOnIntegerOverflow=on  InputSameDT=on
  J : Outport
  wires:
  Selector1/1 -> Jacobian of 2D point/2(Z)
  Selector/1 -> Jacobian of 2D point/1(s)
  Jacobian of 2D point/1(J) -> Assignment/2
  Z/1 -> Selector1/1
  Constant/1 -> Sum/1
  Sum/1 -> Mux/1
  Gain1/1 -> Sum/2, Mux/2
  For Iterator/1 -> Selector1/2, Gain1/1
  Mux/1 -> Assignment/3, Selector/2
  01x6/1 -> Product/2
  Product/1 -> Assignment/1
  Assignment/1 -> J/1
  n/1 -> For Iterator/1
  s/1 -> Selector/1, Product/1

== system vs/Pose/Frame motion/Differential ==
  iTj : Inport
  Vj : Inport  Port=2
  Constant : Constant  Value=[0 0 0 0]  VectorParams1D=off
  Matrix Concatenation : simulink/Math Operations/Matrix Concatenation  numInports=2  catMethod=Horizontal
  Matrix Concatenation1 : simulink/Math Operations/Matrix Concatenation  numInports=2  catMethod=Vertical
  Product : Product  Multiplication=Matrix(*)  SaturateOnIntegerOverflow=on  InputSameDT=on
  Signal Specification : simulink/Signal Attributes/Signal Specification  D=[4 4]  Ts=-1  DataType=auto  OutDataType=sfix(16)  OutScaling=2^0
      settings: SignalType=auto  SamplingMode=auto
  Signal Specification1 : simulink/Signal Attributes/Signal Specification  D=[3 4]  Ts=-1  DataType=auto  OutDataType=sfix(16)  OutScaling=2^0
      settings: SignalType=auto  SamplingMode=auto
  Signal Specification2 : simulink/Signal Attributes/Signal Specification  Orientation=up  D=[3 3]  Ts=-1  DataType=auto  OutDataType=sfix(16)  OutScaling=2^0
      settings: SignalType=auto  SamplingMode=auto
  Signal Specification3 : simulink/Signal Attributes/Signal Specification  D=[3 1]  Ts=-1  DataType=auto  OutDataType=sfix(16)  OutScaling=2^0
      settings: SignalType=auto  SamplingMode=auto
  skew-sym : vs/Pose/skew-sym  SimViewingDevice=off  DataTypeOverride=UseLocalSettings  MinMaxOverflowLogging=UseLocalSettings
      settings: Permissions=ReadWrite  RTWFcnNameOpts=Auto  RTWFileNameOpts=Auto
  vj : Selector  Elements=[1 2 3]  InputPortWidth=6
  wj : Selector  Elements=[4 5 6]  InputPortWidth=6
  diTj : Outport
  wires:
  Vj/1 -> wj/1, vj/1
  wj/1 -> skew-sym/1
  skew-sym/1 -> Signal Specification2/1
  vj/1 -> Signal Specification3/1
  Matrix Concatenation/1 -> Signal Specification1/1
  Constant/1 -> Matrix Concatenation1/2
  iTj/1 -> Product/1
  Matrix Concatenation1/1 -> Product/2
  Product/1 -> Signal Specification/1
  Signal Specification/1 -> diTj/1
  Signal Specification1/1 -> Matrix Concatenation1/1
  Signal Specification2/1 -> Matrix Concatenation/1
  Signal Specification3/1 -> Matrix Concatenation/2

== system vs/Pose/Frame motion/Motion ==
  iTj(0) : Inport
  diTj : Inport  Port=2
  Integrator : Integrator
  Sum : Sum  Inputs=|++  SaturateOnIntegerOverflow=on  InputSameDT=on
  iTj(t) : Outport
  wires:
  diTj/1 -> Integrator/1
  iTj(0)/1 -> Sum/1
  Integrator/1 -> Sum/2
  Sum/1 -> iTj(t)/1

== system vs/Pose/Inverse/Split ==
  T : Inport
  GetP : Selector  InputType=Matrix  Elements=[1 3]  Rows=-1  Columns=4  InputPortWidth=3
  GetR : Selector  InputType=Matrix  Elements=[1 3]  Rows=-1  Columns=[1 2 3]  InputPortWidth=3
  Matrix Concatenation : simulink3/Signals & Systems/Matrix Concatenation  numInports=2  catMethod=Horizontal
  Matrix Concatenation1 : simulink3/Signals & Systems/Matrix Concatenation  numInports=2  catMethod=Horizontal
  P0 : Constant  Value=[0;0;0;1]  VectorParams1D=off
  RI : Constant  Value=[1 0 0; 0 1 0; 0 0 1; 0 0 0]  VectorParams1D=off
  R : Outport
  P : Outport  Port=2
  wires:
  Matrix Concatenation1/1 -> P/1
  GetP/1 -> Matrix Concatenation1/2
  RI/1 -> Matrix Concatenation1/1
  Matrix Concatenation/1 -> R/1
  P0/1 -> Matrix Concatenation/2
  GetR/1 -> Matrix Concatenation/1
  T/1 -> GetR/1, GetP/1

== system vs/Pose/Pose/Euler-rotation ==
  Product : Product  Multiplication=Matrix(*)  SaturateOnIntegerOverflow=on  InputSameDT=on
  Product1 : Product  Multiplication=Matrix(*)  SaturateOnIntegerOverflow=on  InputSameDT=on
  X-rotation theta : Subsystem  mask{phi=theta}
      mask prompts: phi "Angle"
      mask help: Transformation of a pure rotation around the x-axis.
  Z-rotation phi : Subsystem  mask{phi=phi}
      mask prompts: phi "Angle"
      mask help: Transformation of a pure rotation around the z-axis.
  Z-rotation psi : Subsystem  mask{phi=psi}
      mask prompts: phi "Angle"
      mask help: Transformation of a pure rotation around the z-axis.
  T : Outport
  wires:
  Z-rotation psi/1(T) -> Product1/2
  Product/1 -> Product1/1
  X-rotation theta/1(T) -> Product/2
  Z-rotation phi/1(T) -> Product/1
  Product1/1 -> T/1

== system vs/Pose/Pose/RPY-rotation ==
  Product : Product  Multiplication=Matrix(*)  SaturateOnIntegerOverflow=on  InputSameDT=on
  Product1 : Product  Multiplication=Matrix(*)  SaturateOnIntegerOverflow=on  InputSameDT=on
  X-rotation psi : Subsystem  mask{phi=psi}
      mask prompts: phi "Angle"
      mask help: Transformation of a pure rotation around the x-axis.
  Y-rotation theta : Subsystem  mask{phi=theta}
      mask prompts: phi "Angle"
      mask help: Transformation of a pure rotation around the y-axis.
  Z-rotation phi : Subsystem  mask{phi=phi}
      mask prompts: phi "Angle"
      mask help: Transformation of a pure rotation around the z-axis.
  T : Outport
  wires:
  X-rotation psi/1(T) -> Product1/2
  Product/1 -> Product1/1
  Y-rotation theta/1(T) -> Product/2
  Z-rotation phi/1(T) -> Product/1
  Product1/1 -> T/1

== system vs/Pose/Pose/Translation ==
  Constant : Constant  Value=[1 0 0 x;0 1 0 y; 0 0 1 z; 0 0 0 1]  VectorParams1D=off
  T : Outport
  wires:
  Constant/1 -> T/1

== system vs/Pose/Pose2Putheta/Subsystem ==
  sx : Inport
  ny : Inport  Port=2
  az : Inport  Port=3
  Constant : Constant  Orientation=up
  Gain : Gain  Gain=0.5  SaturateOnIntegerOverflow=on
  Sum : Sum  Inputs=|+++-  SaturateOnIntegerOverflow=on  InputSameDT=on
  ctheta : Outport
  wires:
  az/1 -> Sum/3
  Gain/1 -> ctheta/1
  ny/1 -> Sum/2
  sx/1 -> Sum/1
  Sum/1 -> Gain/1
  Constant/1 -> Sum/4

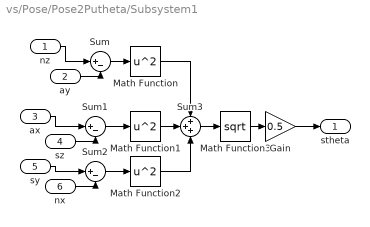
== system vs/Pose/Pose2Putheta/Subsystem1 ==
  nz : Inport
  ay : Inport  Port=2
  ax : Inport  Port=3
  sz : Inport  Port=4
  sy : Inport  Port=5
  nx : Inport  Port=6
  Gain : Gain  Gain=0.5  SaturateOnIntegerOverflow=on
  Math Function : Math  Operator=square
  Math Function1 : Math  Operator=square
  Math Function2 : Math  Operator=square
  Math Function3 : Math  Operator=sqrt
  Sum : Sum  Inputs=|+-  SaturateOnIntegerOverflow=on  InputSameDT=on
  Sum1 : Sum  Inputs=|+-  SaturateOnIntegerOverflow=on  InputSameDT=on
  Sum2 : Sum  Inputs=|+-  SaturateOnIntegerOverflow=on  InputSameDT=on
  Sum3 : Sum  Inputs=+++  SaturateOnIntegerOverflow=on  InputSameDT=on
  stheta : Outport
  wires:
  nx/1 -> Sum2/2
  sy/1 -> Sum2/1
  sz/1 -> Sum1/2
  Gain/1 -> stheta/1
  ax/1 -> Sum1/1
  ay/1 -> Sum/2
  nz/1 -> Sum/1
  Math Function3/1 -> Gain/1
  Sum3/1 -> Math Function3/1
  Math Function2/1 -> Sum3/3
  Math Function1/1 -> Sum3/2
  Math Function/1 -> Sum3/1
  Sum1/1 -> Math Function1/1
  Sum2/1 -> Math Function2/1
  Sum/1 -> Math Function/1

== system vs/Pose/Pose2Putheta/Subsystem2 ==
  ct : Inport
  st : Inport  Port=2
  Trigonometric Function : Trigonometry  Operator=atan2
  theta : Outport
  wires:
  st/1 -> Trigonometric Function/1
  Trigonometric Function/1 -> theta/1
  ct/1 -> Trigonometric Function/2

== system vs/Pose/ScrewTrMat/Split ==
  T : Inport
  GetP : Selector  InputType=Matrix  Elements=[1 3]  Rows=-1  Columns=4  InputPortWidth=3
  GetR : Selector  InputType=Matrix  Elements=[1 3]  Rows=-1  Columns=[1 2 3]  InputPortWidth=3
  Matrix Concatenation : simulink3/Signals & Systems/Matrix Concatenation  numInports=2  catMethod=Horizontal
  Matrix Concatenation1 : simulink3/Signals & Systems/Matrix Concatenation  numInports=2  catMethod=Horizontal
  P0 : Constant  Value=[0;0;0;1]  VectorParams1D=off
  RI : Constant  Value=[1 0 0; 0 1 0; 0 0 1; 0 0 0]  VectorParams1D=off
  R : Outport
  P : Outport  Port=2
  wires:
  Matrix Concatenation1/1 -> P/1
  GetP/1 -> Matrix Concatenation1/2
  RI/1 -> Matrix Concatenation1/1
  Matrix Concatenation/1 -> R/1
  P0/1 -> Matrix Concatenation/2
  GetR/1 -> Matrix Concatenation/1
  T/1 -> GetR/1, GetP/1

== system vs/Camera/Pose estimation/While Iterator Subsystem/J ==
  a : Inport
  b : Inport  Port=2
  Ie1 : Product  Multiplication=Matrix(*)  SaturateOnIntegerOverflow=on  InputSameDT=on
  skew-sym : vs/Pose/skew-sym  SimViewingDevice=off  DataTypeOverride=UseLocalSettings  MinMaxOverflowLogging=UseLocalSettings
      settings: Permissions=ReadWrite  RTWFcnNameOpts=Auto  RTWFileNameOpts=Auto
  axb : Outport
  wires:
  skew-sym/1 -> Ie1/1
  a/1 -> skew-sym/1
  Ie1/1 -> axb/1
  b/1 -> Ie1/2

== system vs/Camera/Pose estimation/While Iterator Subsystem/K ==
  a : Inport
  b : Inport  Port=2
  Ie1 : Product  Multiplication=Matrix(*)  SaturateOnIntegerOverflow=on  InputSameDT=on
  skew-sym : vs/Pose/skew-sym  SimViewingDevice=off  DataTypeOverride=UseLocalSettings  MinMaxOverflowLogging=UseLocalSettings
      settings: Permissions=ReadWrite  RTWFcnNameOpts=Auto  RTWFileNameOpts=Auto
  axb : Outport
  wires:
  skew-sym/1 -> Ie1/1
  a/1 -> skew-sym/1
  Ie1/1 -> axb/1
  b/1 -> Ie1/2

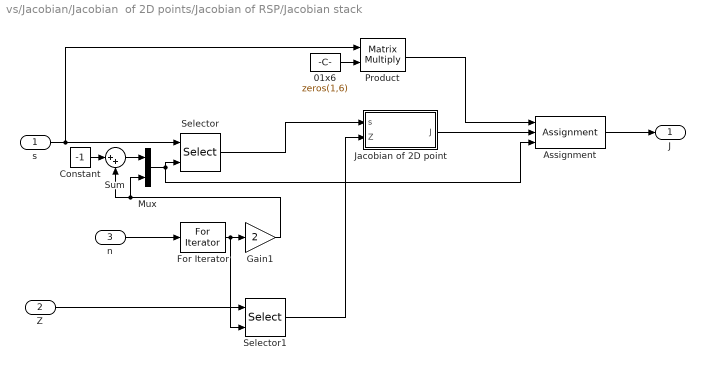
== system vs/Jacobian/Jacobian  of 2D points/Jacobian of RSP/Jacobian stack ==
  s : Inport
  Z : Inport  Port=2
  n : Inport  Port=3
  01x6 : Constant  Value=zeros(1,6)  VectorParams1D=off
  Assignment : Assignment  InputType=Matrix  RowSrc=External  Columns=-1
  Constant : Constant  Value=-1
  For Iterator : ForIterator  IterationSource=external  OutputDataType=double
  Gain1 : Gain  Gain=2  SaturateOnIntegerOverflow=on
  Jacobian of 2D point : Subsystem
  Mux : Mux  Inputs=2
  Product : Product  Multiplication=Matrix(*)  SaturateOnIntegerOverflow=on  InputSameDT=on
  Selector : Selector  InputType=Matrix  ElementSrc=External  Elements=[1 3]  RowSrc=External  Columns=-1  InputPortWidth=3
  Selector1 : Selector  InputType=Matrix  ElementSrc=External  Elements=[1 3]  RowSrc=External  Columns=-1  InputPortWidth=3
  Sum : Sum  Inputs=|++  SaturateOnIntegerOverflow=on  InputSameDT=on
  J : Outport
  wires:
  Selector1/1 -> Jacobian of 2D point/2(Z)
  Selector/1 -> Jacobian of 2D point/1(s)
  Jacobian of 2D point/1(J) -> Assignment/2
  Z/1 -> Selector1/1
  Constant/1 -> Sum/1
  Sum/1 -> Mux/1
  Gain1/1 -> Sum/2, Mux/2
  For Iterator/1 -> Selector1/2, Gain1/1
  Mux/1 -> Assignment/3, Selector/2
  01x6/1 -> Product/2
  Product/1 -> Assignment/1
  Assignment/1 -> J/1
  n/1 -> For Iterator/1
  s/1 -> Selector/1, Product/1

== system vs/Jacobian/Jacobian of 3D points/Jacobian stack/Jacobian of 3D point ==
  s : Inport
  -I3 : Constant  Value=-eye(3)  VectorParams1D=off
  Matrix Concatenation : simulink3/Signals & Systems/Matrix Concatenation  numInports=2  catMethod=Horizontal
  sk(P) : Subsystem
  J : Outport
  wires:
  Matrix Concatenation/1 -> J/1
  s/1 -> sk(P)/1(v)
  sk(P)/1(sk(v)) -> Matrix Concatenation/2
  -I3/1 -> Matrix Concatenation/1

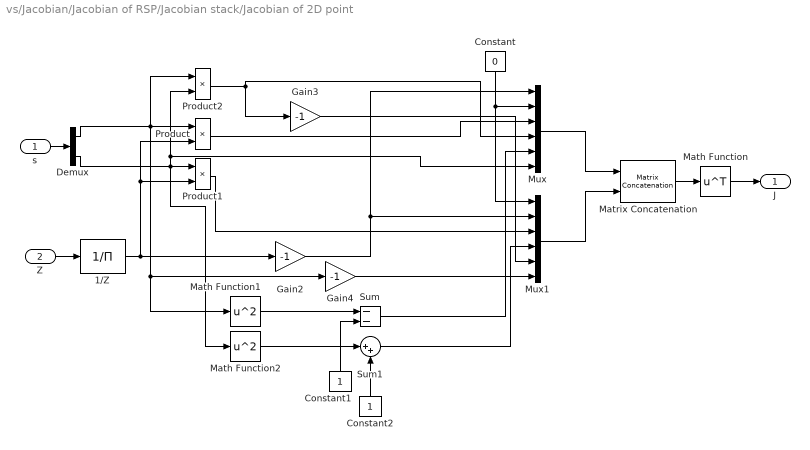
== system vs/Jacobian/Jacobian of RSP/Jacobian stack/Jacobian of 2D point ==
  s : Inport
  Z : Inport  Port=2
  1/Z : Product  Inputs=/  SaturateOnIntegerOverflow=on  InputSameDT=on
  Constant : Constant  Orientation=down  Value=0
  Constant1 : Constant  Orientation=up
  Constant2 : Constant  Orientation=up
  Demux : Demux  Outputs=2
  Gain2 : Gain  Gain=-1  SaturateOnIntegerOverflow=on
  Gain3 : Gain  Gain=-1  SaturateOnIntegerOverflow=on
  Gain4 : Gain  Gain=-1  SaturateOnIntegerOverflow=on
  Math Function : Math  Operator=transpose
  Math Function1 : Math  Operator=square
  Math Function2 : Math  Operator=square
  Matrix Concatenation : simulink3/Signals & Systems/Matrix Concatenation  numInports=2  catMethod=Horizontal
  Mux : Mux  Inputs=6
  Mux1 : Mux  Inputs=6
  Product : Product  SaturateOnIntegerOverflow=on  InputSameDT=on
  Product1 : Product  SaturateOnIntegerOverflow=on  InputSameDT=on
  Product2 : Product  SaturateOnIntegerOverflow=on  InputSameDT=on
  Sum : Sum  Inputs=--  SaturateOnIntegerOverflow=on  InputSameDT=on
  Sum1 : Sum  Inputs=|++  SaturateOnIntegerOverflow=on  InputSameDT=on
  J : Outport
  wires:
  Sum1/1 -> Mux1/4
  Sum/1 -> Mux/5
  Constant2/1 -> Sum1/2
  Constant1/1 -> Sum/2
  Math Function2/1 -> Sum1/1
  Math Function1/1 -> Sum/1
  Product2/1 -> Mux/4, Gain3/1
  Product1/1 -> Mux1/3
  Product/1 -> Mux/3
  Constant/1 -> Mux1/1, Mux/2
  Math Function/1 -> J/1
  Matrix Concatenation/1 -> Math Function/1
  Mux1/1 -> Matrix Concatenation/2
  Mux/1 -> Matrix Concatenation/1
  1/Z/1 -> Product1/2, Product/2, Gain2/1
  Z/1 -> 1/Z/1
  s/1 -> Demux/1
  Demux/1 -> Math Function1/1, Gain4/1, Product2/1, Product/1
  Demux/2 -> Math Function2/1, Product2/2, Mux/6, Product1/1
  Gain2/1 -> Mux1/2, Mux/1
  Gain3/1 -> Mux1/5
  Gain4/1 -> Mux1/6

== system vs/Pose/Pose/Euler-rotation/X-rotation theta ==
  Constant : Constant  Value=[1 0 0 0; 0 cos(phi) -sin(phi) 0; 0 sin(phi) cos(phi) 0; 0 0 0 1]  VectorParams1D=off
  T : Outport
  wires:
  Constant/1 -> T/1

== system vs/Pose/Pose/Euler-rotation/Z-rotation phi ==
  Constant : Constant  Value=[cos(phi) -sin(phi) 0 0; sin(phi) cos(phi) 0 0; 0 0 1 0; 0 0 0 1]  VectorParams1D=off
  T : Outport
  wires:
  Constant/1 -> T/1

== system vs/Pose/Pose/Euler-rotation/Z-rotation psi ==
  Constant : Constant  Value=[cos(phi) -sin(phi) 0 0; sin(phi) cos(phi) 0 0; 0 0 1 0; 0 0 0 1]  VectorParams1D=off
  T : Outport
  wires:
  Constant/1 -> T/1

== system vs/Pose/Pose/RPY-rotation/X-rotation psi ==
  Constant : Constant  Value=[1 0 0 0; 0 cos(phi) -sin(phi) 0; 0 sin(phi) cos(phi) 0; 0 0 0 1]  VectorParams1D=off
  T : Outport
  wires:
  Constant/1 -> T/1

== system vs/Pose/Pose/RPY-rotation/Y-rotation theta ==
  Constant : Constant  Value=[cos(phi) 0 sin(phi) 0; 0 1 0 0; -sin(phi) 0 cos(phi) 0; 0 0 0 1]  VectorParams1D=off
  T : Outport
  wires:
  Constant/1 -> T/1

== system vs/Pose/Pose/RPY-rotation/Z-rotation phi ==
  Constant : Constant  Value=[cos(phi) -sin(phi) 0 0; sin(phi) cos(phi) 0 0; 0 0 1 0; 0 0 0 1]  VectorParams1D=off
  T : Outport
  wires:
  Constant/1 -> T/1

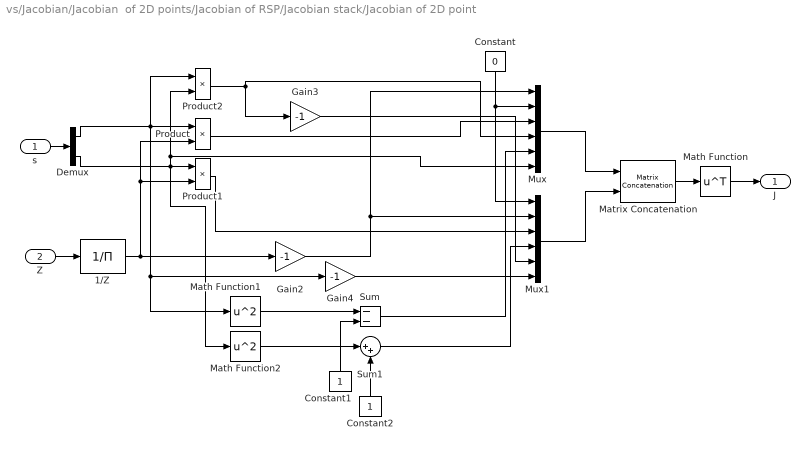
== system vs/Jacobian/Jacobian  of 2D points/Jacobian of RSP/Jacobian stack/Jacobian of 2D point ==
  s : Inport
  Z : Inport  Port=2
  1/Z : Product  Inputs=/  SaturateOnIntegerOverflow=on  InputSameDT=on
  Constant : Constant  Orientation=down  Value=0
  Constant1 : Constant  Orientation=up
  Constant2 : Constant  Orientation=up
  Demux : Demux  Outputs=2
  Gain2 : Gain  Gain=-1  SaturateOnIntegerOverflow=on
  Gain3 : Gain  Gain=-1  SaturateOnIntegerOverflow=on
  Gain4 : Gain  Gain=-1  SaturateOnIntegerOverflow=on
  Math Function : Math  Operator=transpose
  Math Function1 : Math  Operator=square
  Math Function2 : Math  Operator=square
  Matrix Concatenation : simulink3/Signals & Systems/Matrix Concatenation  numInports=2  catMethod=Horizontal
  Mux : Mux  Inputs=6
  Mux1 : Mux  Inputs=6
  Product : Product  SaturateOnIntegerOverflow=on  InputSameDT=on
  Product1 : Product  SaturateOnIntegerOverflow=on  InputSameDT=on
  Product2 : Product  SaturateOnIntegerOverflow=on  InputSameDT=on
  Sum : Sum  Inputs=--  SaturateOnIntegerOverflow=on  InputSameDT=on
  Sum1 : Sum  Inputs=|++  SaturateOnIntegerOverflow=on  InputSameDT=on
  J : Outport
  wires:
  Sum1/1 -> Mux1/4
  Sum/1 -> Mux/5
  Constant2/1 -> Sum1/2
  Constant1/1 -> Sum/2
  Math Function2/1 -> Sum1/1
  Math Function1/1 -> Sum/1
  Product2/1 -> Mux/4, Gain3/1
  Product1/1 -> Mux1/3
  Product/1 -> Mux/3
  Constant/1 -> Mux1/1, Mux/2
  Math Function/1 -> J/1
  Matrix Concatenation/1 -> Math Function/1
  Mux1/1 -> Matrix Concatenation/2
  Mux/1 -> Matrix Concatenation/1
  1/Z/1 -> Product1/2, Product/2, Gain2/1
  Z/1 -> 1/Z/1
  s/1 -> Demux/1
  Demux/1 -> Math Function1/1, Gain4/1, Product2/1, Product/1
  Demux/2 -> Math Function2/1, Product2/2, Mux/6, Product1/1
  Gain2/1 -> Mux1/2, Mux/1
  Gain3/1 -> Mux1/5
  Gain4/1 -> Mux1/6

== system vs/Jacobian/Jacobian of 3D points/Jacobian stack/Jacobian of 3D point/sk(P) ==
  v : Inport
  Constant : Constant  Value=[0 0 0; 0 0 1; 0 -1 0]  VectorParams1D=off
  Constant1 : Constant  Value=[0 0 -1; 0 0 0; 1 0 0]  VectorParams1D=off
  Constant2 : Constant  Value=[0 1 0; -1 0 0; 0 0 0]  VectorParams1D=off
  Matrix Concatenation : simulink3/Signals & Systems/Matrix Concatenation  numInports=3  catMethod=Horizontal
  Product : Product  Multiplication=Matrix(*)  SaturateOnIntegerOverflow=on  InputSameDT=on
  Product1 : Product  Multiplication=Matrix(*)  SaturateOnIntegerOverflow=on  InputSameDT=on
  Product2 : Product  Multiplication=Matrix(*)  SaturateOnIntegerOverflow=on  InputSameDT=on
  sk(v) : Outport
  wires:
  Constant/1 -> Product/1
  v/1 -> Product/2, Product1/2, Product2/2
  Matrix Concatenation/1 -> sk(v)/1
  Product/1 -> Matrix Concatenation/1
  Constant1/1 -> Product1/1
  Constant2/1 -> Product2/1
  Product1/1 -> Matrix Concatenation/2
  Product2/1 -> Matrix Concatenation/3
